simulink model "Lab_2_Simulink"  (R2023b)
settings: Solver=VariableStepAuto  StartTime=0.0  StopTime=inf  RelTol=1e-3
undefined symbols (not defined in the file or in its folder): CR, LF
libraries: instrumentseriallib x3
settings Model: Creator=blake  LastModifiedBy=blake

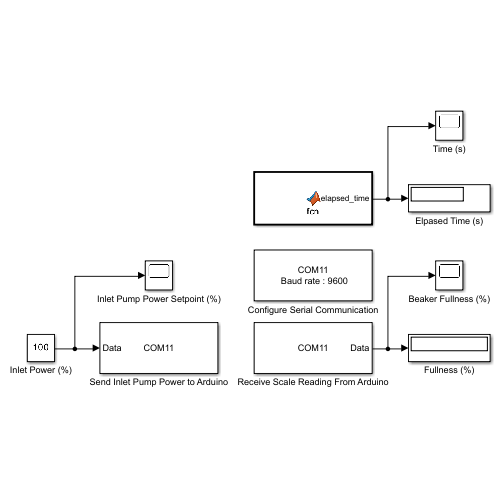
[thumbnail: Simulink's stored preview of the top-level diagram]
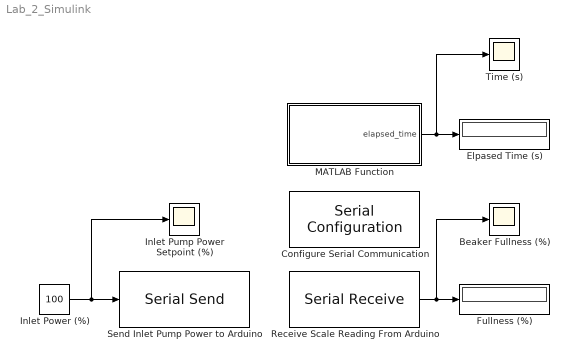
== system Lab_2_Simulink ==
  Beaker Fullness (%) : Scope
  Configure Serial Communication : instrumentseriallib/Serial Configuration  Priority=-200000  PortSel=COM11  Port=COM11  ComPort=COM11  BaudRate=9600  DataBits=8  Parity=none  StopBits=1  ByteOrder=little-endian  FlowControl=none  Timeout=1  SimulateUsing=Interpreted execution  BlockInModel=on  aMode=1
  Elpased Time (s) : Display
  Fullness (%) : Display
  Inlet Power (%) : Constant  Value=100  OutDataTypeStr=single  SampleTime=0.05
  Inlet Pump Power Setpoint (%) : Scope
  MATLAB Function : MATLAB Function  TreatAsAtomicUnit=on
  Receive Scale Reading From Arduino : instrumentseriallib/Serial Receive  Priority=1  PortSel=COM11  Port=COM11  ComPort=COM11  DataType=single  SaveDataType=uint8  ToggleHeader=off  Header=[]  DataSize=1  ToggleTerminator=on  Terminator=CR/LF ('\r\n')  CustomTerminator=[]  InputFormat=Column major  ToggleDataSize=on  EnableBlockingMode=on  ActionDataUnavailable=Output last received value  ActionWhenDataUnavailable=Output last received value  CustomValue=0  SampleTime=0.01  SimulateUsing=Interpreted execution  BlockInModel=on  aMode=1
  Send Inlet Pump Power to Arduino : instrumentseriallib/Serial Send  Priority=1  PortSel=COM11  Port=COM11  ComPort=COM11  Header=[]  Terminator=CR/LF ('\r\n')  CustomTerminator=[]  EnableBlockingMode=on  SimulateUsing=Interpreted execution  BlockInModel=on  aMode=1
  Time (s) : Scope
  wires:
  Receive Scale Reading From Arduino/1 -> Fullness (%)/1, Beaker Fullness (%)/1
  Inlet Power (%)/1 -> Inlet Pump Power Setpoint (%)/1, Send Inlet Pump Power to Arduino/1
  MATLAB Function/1(elapsed_time) -> Time (s)/1, Elpased Time (s)/1

== matlab function Lab_2_Simulink/MATLAB Function ==
  data: elapsed_time output
function elapsed_time = fcn()
    persistent startTime; % persistent variable to store the start time
    
    if isempty(startTime) % check if start_time is empty
        startTime = now;  % initialize start_time with the current time
    end
    
    elapsedDays = now - startTime; % calculate elapsed time in days since start_time
    
    elapsed_time = elapsedDays * 86400; %  convert elapsed time from days to seconds
end
